simulink model "nonLinearised_n9960210"  (R2021a)
settings: Solver=ode14x  StartTime=0.0  StopTime=300  RelTol=1e-3
values from neighbouring files (symbols this model uses):
  A = [0 1 0 ... (first row only)    [main_n9960210_plotall.m]
  a = constant(5)    [main_n9960210_plotall.m]
  alpha = constant(6)    [main_n9960210_plotall.m]
  B = [0 ... (first row only)    [main_n9960210_plotall.m]
  C = [1 0 0]    [main_n9960210_plotall.m]
  controller_enabled = 1    [main_n9960210_plotall.m]
  g = constant(4)    [main_n9960210_plotall.m]
  k = constant(3)    [main_n9960210_plotall.m]
  L = place(A', C', p)'    [main_n9960210_plotall.m]
  L0 = constant(7)    [main_n9960210_plotall.m]
  m = constant(1)    [main_n9960210_plotall.m]
  m0 = constant(2)    [main_n9960210_plotall.m]
  R = 1    [main_n9960210_plotall.m]
  u_bar = 1    [main_n9960210_plotall.m]
  use_state_variables = 1    [main_n9960210_plotall.m]
  x0 = [1.5 0 0]    [main_n9960210_plotall.m]
  x_bar = [2*u_bar-1 ... (first row only)    [main_n9960210_plotall.m]
undefined symbols (not defined in the file or in its folder): K
settings Model: Creator=isaac  LastModifiedBy=isaac

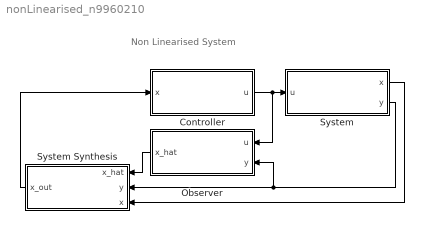
== system nonLinearised_n9960210 ==
  note: Non Linearised System
  Controller : Subsystem
  Observer : Subsystem
  System : Subsystem
  System Synthesis : Subsystem
  wires:
  System/2(y) -> Observer/2(y), System Synthesis/2(y)
  Controller/1(u) -> Observer/1(u), System/1(u)
  System/1(x) -> System Synthesis/3(x)
  Observer/1(x_hat) -> System Synthesis/1(x_hat)
  System Synthesis/1(x_out) -> Controller/1(x)

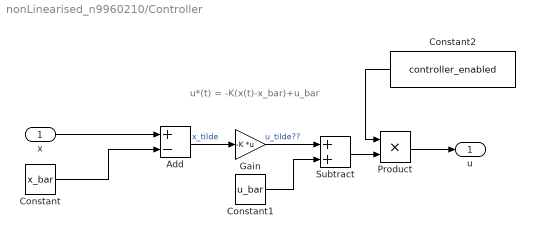
== system nonLinearised_n9960210/Controller ==
  note: u*(t) = -K(x(t)-x_bar)+u_bar
  x : Inport
  Add : Sum  Inputs=+-
  Constant : Constant  Value=x_bar
  Constant1 : Constant  Value=u_bar
  Constant2 : Constant  Value=controller_enabled
  Gain : Gain  Gain=-K  Multiplication=Matrix(K*u)
  Product : Product
  Subtract : Sum
  u : Outport
  wires:
  Add/1 -> Gain/1  "x_tilde"
  Constant/1 -> Add/2
  x/1 -> Add/1
  Constant1/1 -> Subtract/2
  Gain/1 -> Subtract/1  "u_tilde??"
  Subtract/1 -> Product/2
  Constant2/1 -> Product/1
  Product/1 -> u/1

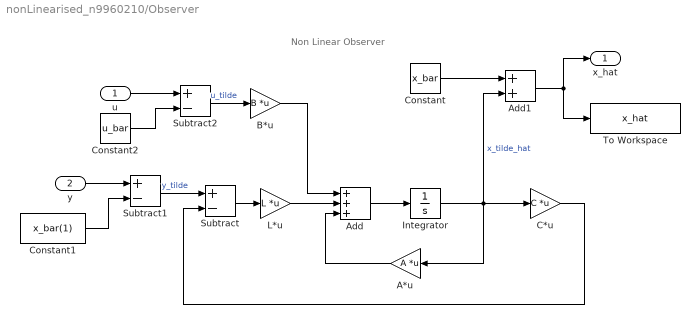
== system nonLinearised_n9960210/Observer ==
  note: Non Linear Observer
  u : Inport
  y : Inport  Port=2
  A*u : Gain  Gain=A  Multiplication=Matrix(K*u)
  Add : Sum  Inputs=+++
  Add1 : Sum
  B*u : Gain  Gain=B  Multiplication=Matrix(K*u)
  C*u : Gain  Gain=C  Multiplication=Matrix(K*u)
  Constant : Constant  Value=x_bar
  Constant1 : Constant  Value=x_bar(1)
  Constant2 : Constant  Value=u_bar
  Integrator : Integrator  InitialCondition=x0-x_bar'
  L*u : Gain  Gain=L  Multiplication=Matrix(K*u)
  Subtract : Sum  Inputs=+-
  Subtract1 : Sum  Inputs=+-
  Subtract2 : Sum  Inputs=+-
  To Workspace : ToWorkspace  VariableName=x_hat  SampleTime=-1
  x_hat : Outport
  wires:
  Constant1/1 -> Subtract1/2
  L*u/1 -> Add/2
  Add/1 -> Integrator/1
  A*u/1 -> Add/3
  Constant/1 -> Add1/1
  y/1 -> Subtract1/1
  Subtract1/1 -> Subtract/1  "y_tilde"
  Subtract/1 -> L*u/1
  Add1/1 -> To Workspace/1, x_hat/1
  Integrator/1 -> Add1/2, C*u/1, A*u/1  "x_tilde_hat"
  C*u/1 -> Subtract/2
  B*u/1 -> Add/1
  u/1 -> Subtract2/1
  Subtract2/1 -> B*u/1  "u_tilde"
  Constant2/1 -> Subtract2/2

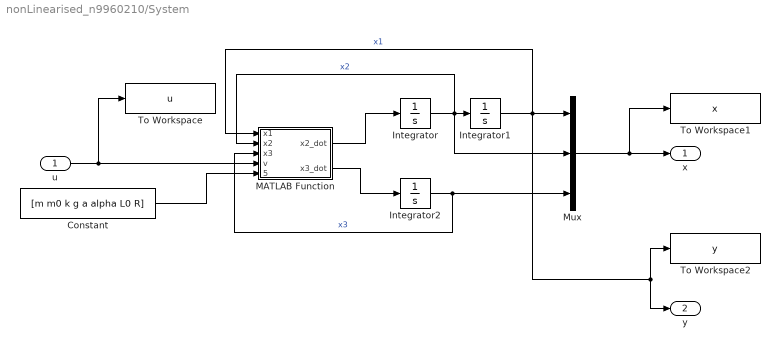
== system nonLinearised_n9960210/System ==
  u : Inport
  Constant : Constant  Value=[m m0 k g a alpha L0 R]
  Integrator : Integrator  InitialCondition=x0(2)
  Integrator1 : Integrator  InitialCondition=x0(1)
  Integrator2 : Integrator  InitialCondition=x0(3)
  MATLAB Function : MATLAB Function  TreatAsAtomicUnit=on
  Mux : Mux  Inputs=3
  To Workspace : ToWorkspace  VariableName=u  SampleTime=-1
  To Workspace1 : ToWorkspace  VariableName=x  SampleTime=-1
  To Workspace2 : ToWorkspace  VariableName=y  SampleTime=-1
  x : Outport
  y : Outport  Port=2
  wires:
  Integrator2/1 -> MATLAB Function/3(x3), Mux/3  "x3"
  Mux/1 -> To Workspace1/1, x/1
  Integrator1/1 -> To Workspace2/1, y/1, MATLAB Function/1(x1), Mux/1  "x1"
  MATLAB Function/2(x3_dot) -> Integrator2/1
  u/1 -> To Workspace/1, MATLAB Function/4(v)
  Integrator/1 -> Integrator1/1, Mux/2, MATLAB Function/2(x2)  "x2"
  Constant/1 -> MATLAB Function/5(constant)
  MATLAB Function/1(x2_dot) -> Integrator/1

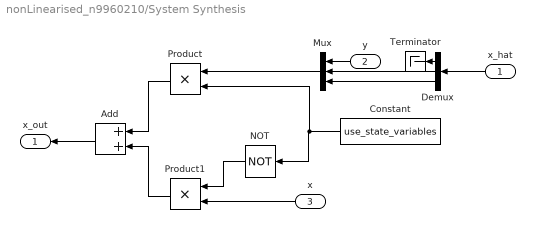
== system nonLinearised_n9960210/System Synthesis ==
  x_hat : Inport
  y : Inport  Port=2
  x : Inport  Port=3
  Add : Sum  Inputs=2
  Constant : Constant  Value=use_state_variables
  Demux : Demux  Outputs=3
  Mux : Mux  Inputs=3
  NOT : Logic  Operator=NOT  IconShape=distinctive  AllPortsSameDT=off  OutDataTypeStr=boolean
  Product : Product
  Product1 : Product
  Terminator : Terminator
  x_out : Outport
  wires:
  Add/1 -> x_out/1
  Product/1 -> Add/1
  Product1/1 -> Add/2
  x/1 -> Product1/2
  NOT/1 -> Product1/1
  Constant/1 -> Product/2, NOT/1
  Mux/1 -> Product/1
  x_hat/1 -> Demux/1
  Demux/3 -> Mux/3
  y/1 -> Mux/1
  Demux/1 -> Terminator/1
  Demux/2 -> Mux/2

== matlab function nonLinearised_n9960210/System/MATLAB Function ==
  data: x1 input; x2 input; x2_dot output; x3 input; v input; constant input; x3_dot output
function [x2_dot, x3_dot] = fcn(x1,x2,x3,v,constant)

m = constant(1);
m0 = constant(2);
k = constant(3);
g = constant(4);
a = constant(5);
alpha = constant(6);
L0 = constant(7);
R = constant(8);

lambda = sqrt(g/a);
b = k/(lambda*m);
beta = lambda*L0/R;
c = m0/m;
I = sqrt(8*alpha*m0*g)/L0;
u = v;
T = beta*(1+1/(1+x1));

x2_dot = -b*x2+1-((4*c*x3^2)/(1+x1)^2);
x3_dot = (1/T)*(-x3+u+((beta*x2*x3)/(1+x1)^2));
